simulink subsystem "ModelBasedArmControl"  (R2023a)
settings: Solver=VariableStepAuto  StartTime=0.0  StopTime=10.0  RelTol=1e-3
undefined symbols (not defined in the file or in its folder): DiscIntNeverNeededParam, jointControlData, nLink
libraries: simulink x1
settings Model: Creator=Andy  LastModifiedBy=Andy
settings OptimizationCC: ReuseModelBlockBuffer=off
settings ModelReferenceCC: EnableRefExpFcnMdlSchedulingChecks=on

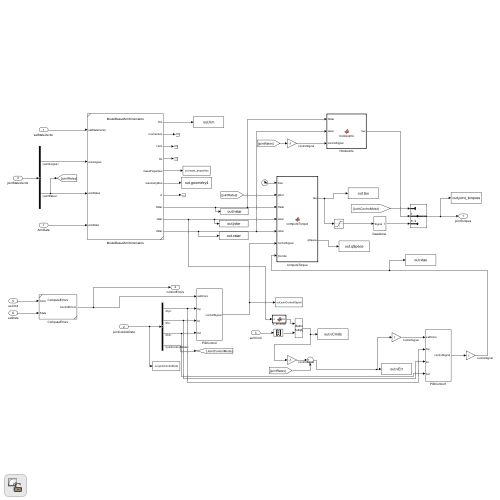
[thumbnail: Simulink's stored preview of the top-level diagram]
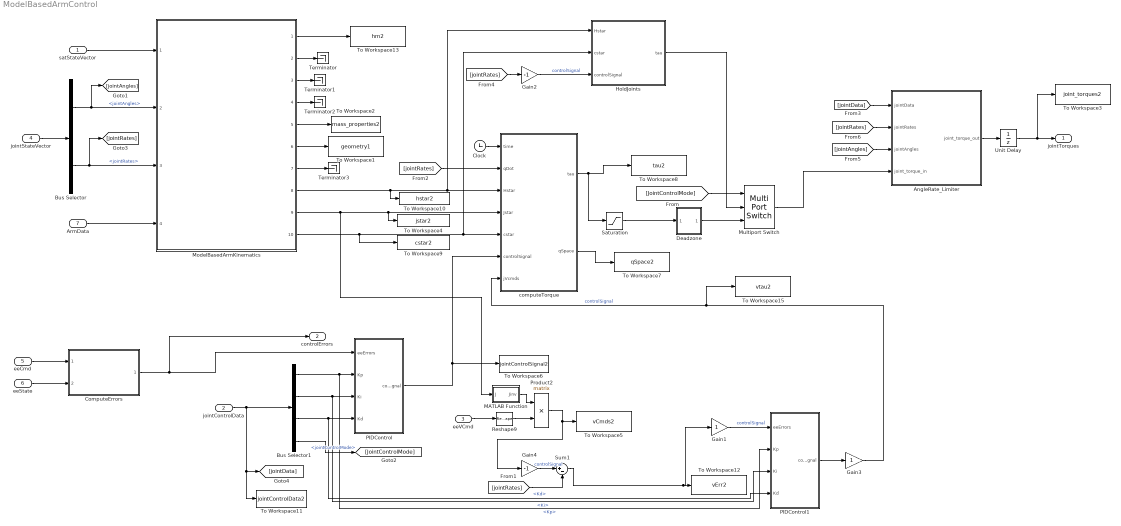
== system ModelBasedArmControl ==
  satStateVector : Inport
  jointControlData : Inport  Port=2
  eeVCmd : Inport  Port=3
  jointStateVector : Inport  Port=4
  eeCmd : Inport  Port=5
  eeState : Inport  Port=6
  ArmData : Inport  Port=7
  AngleRate_Limiter : Subsystem
  Bus Selector : BusSelector  OutputSignals=jointAngles,jointRates
  Bus Selector1 : BusSelector  OutputSignals=Kp,Ki,Kd,jointControlMode
  Clock : Clock
  ComputeErrors : Subsystem  ReferencedSubsystem=ComputeErrors
  "Deadzone " : Subsystem
  Gain1 : Gain
  Gain2 : Gain  Gain=-1
  Gain3 : Gain
  Gain4 : Gain  Gain=-1
  HoldJoints : MATLAB Function
  MATLAB Function : MATLAB Function  TreatAsAtomicUnit=on
  ModelBasedArmKinematics : Subsystem  VariantControl=VSS_ModelBasedArmControl  ReferencedSubsystem=ModelBasedArmKinematics
  Multiport Switch : MultiPortSwitch  Inputs=2  SaturateOnIntegerOverflow=off  InputSameDT=off
  PIDControl : Subsystem
  PIDControl1 : Subsystem
  Product2 : Product  Multiplication=Matrix(*)
  Reshape9 : Reshape  OutputDimensionality=Column vector (2-D)  OutputDimensions=[1,12]
  Saturation : Saturate  UpperLimit=jointControlData.torqueLimit  LowerLimit=-jointControlData.torqueLimit
  Sum1 : Sum  Inputs=|+-
  Terminator{,1..3} (4 alike) : Terminator
  To Workspace1 : ToWorkspace  VariableName=geometry1  SaveFormat=Timeseries  SampleTime=-1
  To Workspace10 : ToWorkspace  VariableName=hstar2  SaveFormat=Timeseries  SampleTime=-1
  To Workspace11 : ToWorkspace  VariableName=jointControlData2  SaveFormat=Timeseries  SampleTime=-1
  To Workspace12 : ToWorkspace  VariableName=vErr2  SaveFormat=Timeseries  SampleTime=-1
  To Workspace13 : ToWorkspace  VariableName=hm2  SaveFormat=Timeseries  SampleTime=-1
  To Workspace15 : ToWorkspace  VariableName=vtau2  SaveFormat=Timeseries  SampleTime=-1
  To Workspace2 : ToWorkspace  VariableName=mass_properties2  SaveFormat=Timeseries  SampleTime=-1
  To Workspace3 : ToWorkspace  VariableName=joint_torques2  SaveFormat=Timeseries  SampleTime=-1
  To Workspace4 : ToWorkspace  VariableName=jstar2  SaveFormat=Timeseries  SampleTime=-1
  To Workspace5 : ToWorkspace  VariableName=vCmds2  SaveFormat=Timeseries  SampleTime=-1
  To Workspace6 : ToWorkspace  VariableName=jointControlSignal2  SaveFormat=Timeseries  SampleTime=-1
  To Workspace7 : ToWorkspace  VariableName=qSpace2  SaveFormat=Timeseries  SampleTime=-1
  To Workspace8 : ToWorkspace  VariableName=tau2  SaveFormat=Timeseries  SampleTime=-1
  To Workspace9 : ToWorkspace  VariableName=cstar2  SaveFormat=Timeseries  SampleTime=-1
  Unit Delay : UnitDelay  SampleTime=-1  HasFrameUpgradeWarning=on
  computeTorque : MATLAB Function
  jointTorques : Outport
  controlErrors : Outport  Port=2
  wires:
  Bus Selector/2 -> ModelBasedArmKinematics/3, [jointRates]  "<jointRates>"
  Bus Selector/1 -> ModelBasedArmKinematics/2, [jointAngles]  "<jointAngles>"
  ArmData/1 -> ModelBasedArmKinematics/4
  eeState/1 -> ComputeErrors/2
  eeCmd/1 -> ComputeErrors/1
  [jointRates] -> Sum1/2
  [jointRates] -> Gain2/1
  [jointRates] -> computeTorque/2(qDot)
  ModelBasedArmKinematics/7 -> Terminator3/1
  ModelBasedArmKinematics/4 -> Terminator2/1
  ModelBasedArmKinematics/3 -> Terminator1/1
  ModelBasedArmKinematics/2 -> Terminator/1
  satStateVector/1 -> ModelBasedArmKinematics/1
  ModelBasedArmKinematics/5 -> To Workspace2/1
  "Deadzone "/1(Out1) -> Multiport Switch/3
  Gain4/1 -> Sum1/1  "controlSignal"
  Gain3/1 -> To Workspace15/1, computeTorque/7(jVcmds)  "controlSignal"
  computeTorque/1(tau) -> Saturation/1, To Workspace8/1
  Gain1/1 -> PIDControl1/1(eeErrors)  "controlSignal"
  jointStateVector/1 -> Bus Selector/1
  ModelBasedArmKinematics/1 -> To Workspace13/1
  PIDControl1/1(controlSignal) -> Gain3/1
  Sum1/1 -> Gain1/1, To Workspace12/1
  Reshape9/1 -> Product2/2
  MATLAB Function/1(Jinv) -> Product2/1
  Product2/1 -> To Workspace5/1, Gain4/1
  eeVCmd/1 -> Reshape9/1
  ComputeErrors/1 -> controlErrors/1, PIDControl/1(eeErrors)
  Gain2/1 -> HoldJoints/3(controlSignal)  "controlSignal"
  ModelBasedArmKinematics/9 -> To Workspace4/1, computeTorque/4(Jstar), MATLAB Function/1(J)
  computeTorque/2(qSpace) -> To Workspace7/1
  PIDControl/1(controlSignal) -> computeTorque/6(controlSignal), To Workspace6/1
  Clock/1 -> computeTorque/1(time)
  HoldJoints/1(tau) -> Multiport Switch/2
  [JointControlMode] -> Multiport Switch/1
  Saturation/1 -> "Deadzone "/1(Signal)
  Bus Selector1/1 -> PIDControl1/2(Kp), PIDControl/2(Kp)  "<Kp>"
  ModelBasedArmKinematics/10 -> HoldJoints/2(cstar), computeTorque/5(cstar), To Workspace9/1
  Bus Selector1/2 -> PIDControl1/3(Ki), PIDControl/3(Ki)  "<Ki>"
  Bus Selector1/3 -> PIDControl1/4(Kd), PIDControl/4(Kd)  "<Kd>"
  ModelBasedArmKinematics/8 -> computeTorque/3(Hstar), HoldJoints/1(Hstar), To Workspace10/1
  ModelBasedArmKinematics/6 -> To Workspace1/1
  jointControlData/1 -> To Workspace11/1, [jointData], Bus Selector1/1
  Bus Selector1/4 -> [JointControlMode]  "<jointControlMode>"
  [jointData] -> AngleRate_Limiter/1(jointData)
  [jointRates] -> AngleRate_Limiter/2(jointRates)
  [jointAngles] -> AngleRate_Limiter/3(jointAngles)
  Multiport Switch/1 -> AngleRate_Limiter/4(joint_torque_in)
  AngleRate_Limiter/1(joint_torque_out) -> Unit Delay/1
  Unit Delay/1 -> jointTorques/1, To Workspace3/1

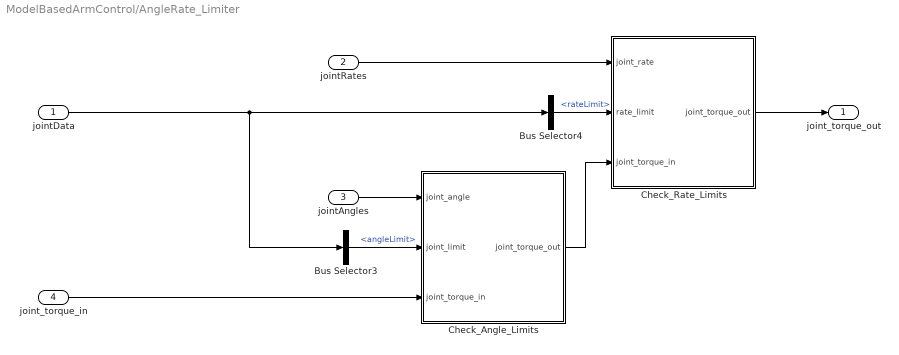
== system ModelBasedArmControl/AngleRate_Limiter ==
  jointData : Inport
  jointRates : Inport  Port=2
  jointAngles : Inport  Port=3
  joint_torque_in : Inport  Port=4
  Bus Selector3 : BusSelector  OutputSignals=angleLimit
  Bus Selector4 : BusSelector  OutputSignals=rateLimit
  Check_Angle_Limits : MATLAB Function
  Check_Rate_Limits : MATLAB Function
  joint_torque_out : Outport
  wires:
  jointRates/1 -> Check_Rate_Limits/1(joint_rate)
  jointAngles/1 -> Check_Angle_Limits/1(joint_angle)
  Check_Rate_Limits/1(joint_torque_out) -> joint_torque_out/1
  joint_torque_in/1 -> Check_Angle_Limits/3(joint_torque_in)
  Bus Selector3/1 -> Check_Angle_Limits/2(joint_limit)  "<angleLimit>"
  Check_Angle_Limits/1(joint_torque_out) -> Check_Rate_Limits/3(joint_torque_in)
  Bus Selector4/1 -> Check_Rate_Limits/2(rate_limit)  "<rateLimit>"
  jointData/1 -> Bus Selector4/1, Bus Selector3/1

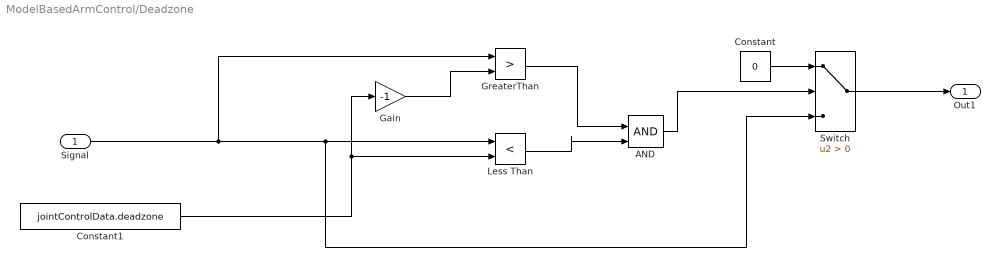
== system ModelBasedArmControl/Deadzone  ==
  Signal : Inport
  AND : Logic  IconShape=distinctive  AllPortsSameDT=off  OutDataTypeStr=boolean
  Constant : Constant  Value=0
  Constant1 : Constant  Value=jointControlData.deadzone
  Gain : Gain  Gain=-1
  GreaterThan : RelationalOperator  Operator=>  OutDataTypeStr=boolean  RndMeth=Simplest  InputSameDT=off
  Less Than : RelationalOperator  Operator=<  OutDataTypeStr=boolean  RndMeth=Simplest  InputSameDT=off
  Switch : Switch  Criteria=u2 > Threshold  SaturateOnIntegerOverflow=off  InputSameDT=off
  Out1 : Outport
  wires:
  Gain/1 -> GreaterThan/2
  GreaterThan/1 -> AND/1
  Constant1/1 -> Less Than/2, Gain/1
  Less Than/1 -> AND/2
  AND/1 -> Switch/2
  Signal/1 -> Switch/3, Less Than/1, GreaterThan/1
  Switch/1 -> Out1/1
  Constant/1 -> Switch/1

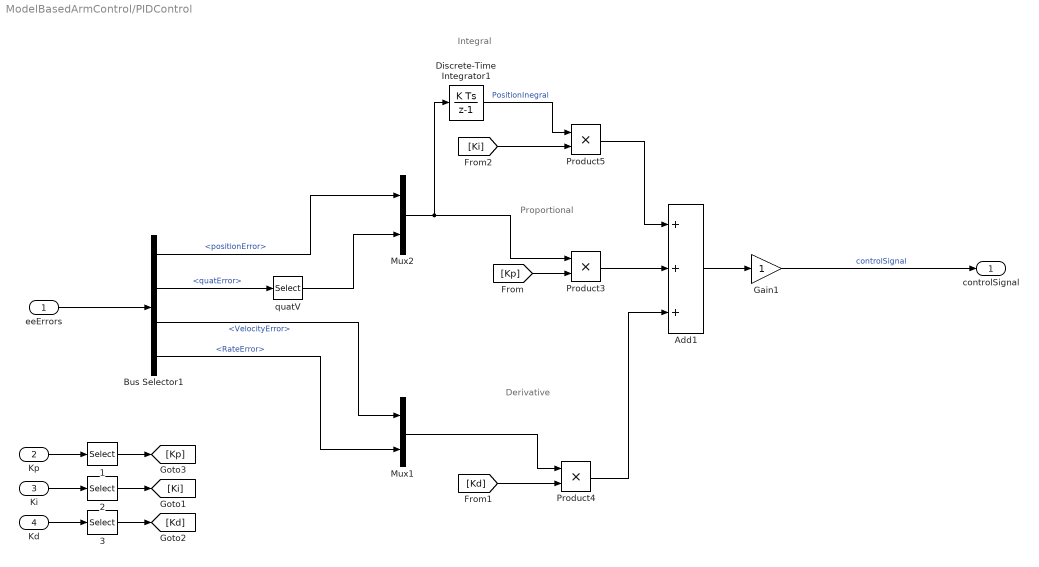
== system ModelBasedArmControl/PIDControl ==
  note: Derivative
  note: Proportional
  note: Integral
  eeErrors : Inport
  Kp : Inport  Port=2
  Ki : Inport  Port=3
  Kd : Inport  Port=4
  1 : Selector  IndexOptions=Index vector (dialog)  Indices=1:6  OutputSizes=1
  2 : Selector  IndexOptions=Index vector (dialog)  Indices=1:6  OutputSizes=1
  3 : Selector  IndexOptions=Index vector (dialog)  Indices=1:6  OutputSizes=1
  Add1 : Sum  Inputs=+++
  Bus Selector1 : BusSelector  OutputSignals=positionError,quatError,VelocityError,RateError
  Discrete-Time Integrator1 : DiscreteIntegrator  SampleTime=-1  ICPrevOutput=DiscIntNeverNeededParam  ICPrevScaledInput=DiscIntNeverNeededParam
  Gain1 : Gain
  Mux1 : Mux  Inputs=2
  Mux2 : Mux  Inputs=2
  Product3 : Product
  Product4 : Product
  Product5 : Product
  quatV : Selector  IndexOptions=Index vector (dialog)  Indices=[2:4]  OutputSizes=1
  controlSignal : Outport
  wires:
  Mux2/1 -> Discrete-Time Integrator1/1, Product3/1
  Discrete-Time Integrator1/1 -> Product5/1  "PositionInegral"
  Product5/1 -> Add1/1
  Gain1/1 -> controlSignal/1  "controlSignal"
  Mux1/1 -> Product4/1
  [Ki] -> Product5/2
  [Kp] -> Product3/2
  [Kd] -> Product4/2
  Add1/1 -> Gain1/1
  Product4/1 -> Add1/3
  Kp/1 -> 1/1
  Kd/1 -> 3/1
  Ki/1 -> 2/1
  Product3/1 -> Add1/2
  eeErrors/1 -> Bus Selector1/1
  Bus Selector1/1 -> Mux2/1  "<positionError>"
  Bus Selector1/2 -> quatV/1  "<quatError>"
  Bus Selector1/3 -> Mux1/1  "<VelocityError>"
  Bus Selector1/4 -> Mux1/2  "<RateError>"
  quatV/1 -> Mux2/2
  1/1 -> [Kp]
  2/1 -> [Ki]
  3/1 -> [Kd]

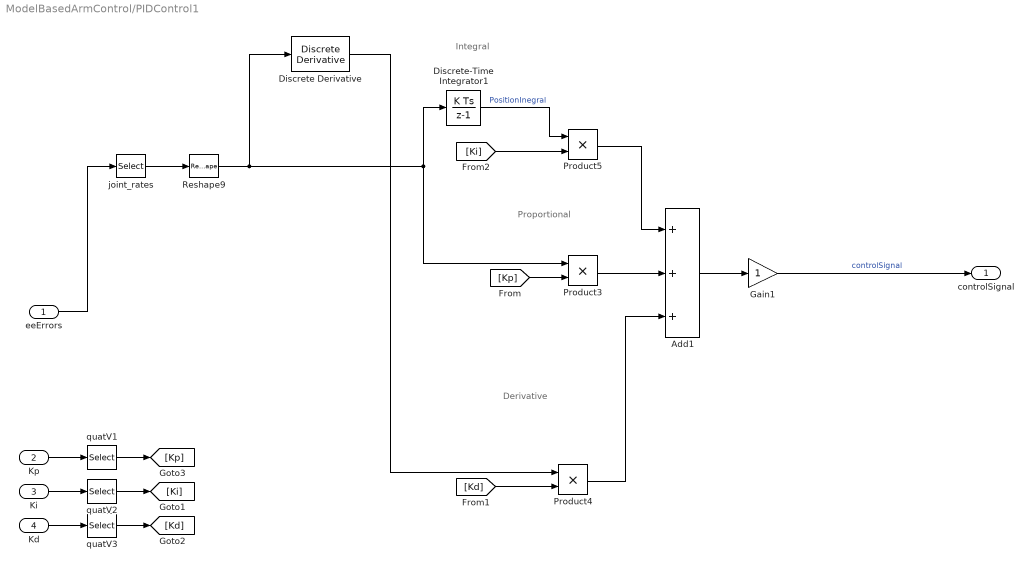
== system ModelBasedArmControl/PIDControl1 ==
  note: Integral
  note: Proportional
  note: Derivative
  eeErrors : Inport
  Kp : Inport  Port=2
  Ki : Inport  Port=3
  Kd : Inport  Port=4
  Add1 : Sum  Inputs=+++
  Discrete Derivative : simulink/Discrete/Discrete Derivative  gainval=1.0  ICPrevScaledInput=0.0  OutMin=[]  OutMax=[]  OutDataType=fixdt(1, 16)  OutScaling=2^-10  DoSatur=off
  Discrete-Time Integrator1 : DiscreteIntegrator  SampleTime=-1  ICPrevOutput=DiscIntNeverNeededParam  ICPrevScaledInput=DiscIntNeverNeededParam
  Gain1 : Gain
  Product3 : Product
  Product4 : Product
  Product5 : Product
  Reshape9 : Reshape  OutputDimensionality=Row vector (2-D)  OutputDimensions=[1,12]
  joint_rates : Selector  IndexOptions=Index vector (dialog)  Indices=1:nLink  OutputSizes=1
  quatV1 : Selector  IndexOptions=Index vector (dialog)  Indices=1:nLink  OutputSizes=1
  quatV2 : Selector  IndexOptions=Index vector (dialog)  Indices=1:nLink  OutputSizes=1
  quatV3 : Selector  IndexOptions=Index vector (dialog)  Indices=1:nLink  OutputSizes=1
  controlSignal : Outport
  wires:
  Product3/1 -> Add1/2
  Ki/1 -> quatV2/1
  Kd/1 -> quatV3/1
  Kp/1 -> quatV1/1
  Product4/1 -> Add1/3
  Add1/1 -> Gain1/1
  [Kd] -> Product4/2
  [Kp] -> Product3/2
  [Ki] -> Product5/2
  Gain1/1 -> controlSignal/1  "controlSignal"
  Product5/1 -> Add1/1
  Discrete-Time Integrator1/1 -> Product5/1  "PositionInegral"
  quatV1/1 -> [Kp]
  quatV2/1 -> [Ki]
  quatV3/1 -> [Kd]
  eeErrors/1 -> joint_rates/1
  joint_rates/1 -> Reshape9/1
  Discrete Derivative/1 -> Product4/1
  Reshape9/1 -> Discrete Derivative/1, Discrete-Time Integrator1/1, Product3/1

== matlab function ModelBasedArmControl/AngleRate_Limiter/Check_Angle_Limits ==
  data: joint_torque_out output; joint_angle input; joint_limit input; joint_torque_in input; NLINKS parameter
function joint_torque_out = Check_Angle_Limits(joint_angle,joint_limit,joint_torque_in,NLINKS)

% The line below broke the signal size back propagation, so instead set
% it to zeros and set each element individually
% joint_torque_out = joint_torque_in; 

joint_torque_out = zeros(NLINKS,1);

% If the current angle is near the limit and the torque continues
% to move that direction, zero it.
for i = 1:NLINKS
    if joint_angle(i) < 0
        % Negative case
        if joint_angle(i)/joint_limit(i,1) > 0.95 && joint_torque_in(i) < 0
            joint_torque_out(i) = 0.0;
        else
            joint_torque_out(i) = joint_torque_in(i);
        end
    else
        % Positive case
        if joint_angle(i)/joint_limit(i,2) > 0.95 && joint_torque_in(i) > 0
            joint_torque_out(i) = 0.0;
        else
            joint_torque_out(i) = joint_torque_in(i);
        end
    end
end

== matlab function ModelBasedArmControl/AngleRate_Limiter/Check_Rate_Limits ==
  data: joint_torque_out output; joint_rate input; rate_limit input; joint_torque_in input; NLINKS parameter
function joint_torque_out = Check_Rate_Limits(joint_rate,rate_limit,joint_torque_in,NLINKS)

% The line below broke the signal size back propagation, so instead set
% it to zeros and set each element individually
% joint_torque_out = joint_torque_in; 

joint_torque_out = zeros(NLINKS,1);

% If the current rate is at or above the limit and the torque command would
% continue to move that direction, zero it.

for i = 1:NLINKS
    if joint_rate(i) < 0
        % Negative case
        if abs(joint_rate(i)) >= rate_limit(i) && joint_torque_in(i) < 0
            joint_torque_out(i) = 0.0;
        else
            joint_torque_out(i) = joint_torque_in(i);
        end
    else
        % Positive case
        if abs(joint_rate(i)) >= rate_limit(i) && joint_torque_in(i) > 0
            joint_torque_out(i) = 0.0;
        else
            joint_torque_out(i) = joint_torque_in(i);
        end
    end
end

== matlab function ModelBasedArmControl/HoldJoints ==
  data: Hstar input; tau output; cstar input; controlSignal input
function tau  = holdJoints(Hstar,cstar,controlSignal)

% Compute joint torques
tau = Hstar*controlSignal - cstar';

== matlab function ModelBasedArmControl/MATLAB Function ==
  data: J input; Jinv output
function Jinv  = J_inverse(J)

Jinv = pinv(J);

== matlab function ModelBasedArmControl/computeTorque ==
  data: time input; qDot input; Hstar input; tau output; Jstar input; cstar input; controlSignal input; jVcmds input; NLINKS parameter; qSpace output
function [tau,qSpace]  = computeTorque(time,qDot,Hstar,Jstar,cstar,controlSignal,jVcmds,NLINKS)

% tau = zeros(NLINKS,1);
%qSpace = zeros(NLINKS,1);
rows = [1 2 6];
% Compute inverse of generalized Jacobian
JstarInv = pinv(Jstar);
% JstarInv = pinv(Jstar(rows,:));

% Transform to joint rates
qSpace = JstarInv*controlSignal';
% qSpace = JstarInv*controlSignal(rows)';

if norm(JstarInv) > 50
    % tau = zeros(NLINKS,1);
    tau = qDot.*0;
else
    
    Cstar = Hstar*(qDot) + cstar';
    
    %tau = 0.1.*Hstar*qSpace + Cstar;
    % Compute joint torques
    tau = Hstar*qSpace + cstar';
    % tau = Hstar*qSpace + Cstar;
    
    tau = Hstar*jVcmds' + Cstar;
end
